simulink library "tqd"  (R2021b)
settings: Solver=VariableStepAuto  StartTime=0.0  StopTime=10.0  RelTol=1e-3
undefined symbols (not defined in the file): ATQD_AfterTqMinGain_X_Deg, ATQD_APSCreepBaseTqD_X_kph, ATQD_APSCreepBaseTqD_Y_Deg, ATQD_APSCreepBaseTqR_X_kph, ATQD_APSCreepBaseTqR_Y_Deg, ATQD_APSCreepIterm_X_kph, ATQD_APSCreepIterm_Y_kph, ATQD_APSCreepPterm_X_kph, ATQD_APSCreepPterm_Y_kph, ATQD_APSDecReq_X_kph, ATQD_APSDecReq_Y_mps2, ATQD_APSDecReqCMD_X_kph, ATQD_APSDecReqTs_X_pct, ATQD_APSDecTimeGain_X_Deg, ATQD_APSDecTimeGain_Y_s, ATQD_APSReqLowSpd_X_Deg, ATQD_AutoHoldReleaseBPS_X_Deg, ATQD_AWDLoadTrqnsGain_X_kg, ATQD_AWDLoadTrqnsGain_Y_pct, ATQD_BOSEnBPSPosn_X_kph, ATQD_BOSMap_X_rpm, ATQD_BOSMap_Y_pct, ATQD_CreepBaseTqD_X_kph, ATQD_CreepBaseTqD_Y_Deg, ATQD_CreepBaseTqR_X_kph, ATQD_CreepBaseTqR_Y_Deg, ATQD_CreepBPSDisPosn_X_Deg, ATQD_CreepBPSDisPosnR_X_Deg, ATQD_CreepBPSEnPosn_X_Deg, ATQD_CreepBPSEnPosnR_X_Deg, ATQD_CreepDeltaTq_X_kph, ATQD_CreepIterm_X_kph, ATQD_CreepIterm_Y_kph, ATQD_CreepItermMaxLimit_X_pct, ATQD_CreepPreloadTime_X_kph, ATQD_CreepPreloadTq_X_kph, ATQD_CreepPreloadTq_Y_s, ATQD_CreepProtTq_X_Deg, ATQD_CreepPterm_X_kph, ATQD_CreepPterm_Y_kph, ATQD_CreepRrTqSpRat_X_rpm, ATQD_CreepRrTqSpRat_Y_Nm, ATQD_CreepTargetSpdD_X_pct, ATQD_CreepTargetSpdR_X_pct, ATQD_ECOTqMapD_X_rpm, ATQD_ECOTqMapD_Y_pct, ATQD_EMTqMapD_X_rpm, ATQD_EMTqMapD_Y_pct, ATQD_EOPDTqMapDCon_X_rpm, ATQD_EOPDTqMapDCon_Y_Deg, ATQD_EscapeModePedTq_X_pct, ATQD_EscapeModePedTq_Y_rpm, ATQD_EscapeModePedTqFr_X_pct, ATQD_EscapeModePedTqFr_Y_rpm, ATQD_EstInitVehWeight_X_c, ATQD_FAfterTqCMDGain_X_rpm, ATQD_FAfterTqCMDGain_Y_pct, ATQD_FrLossMAPLowV_X_rpm, ATQD_FrLossMAPLowV_Y_Nm, ATQD_FrMotActReduce_X_rpm ... (+772)
libraries: simulink x211, hcu_lib x179, tqr x3
(part 9 of 28)

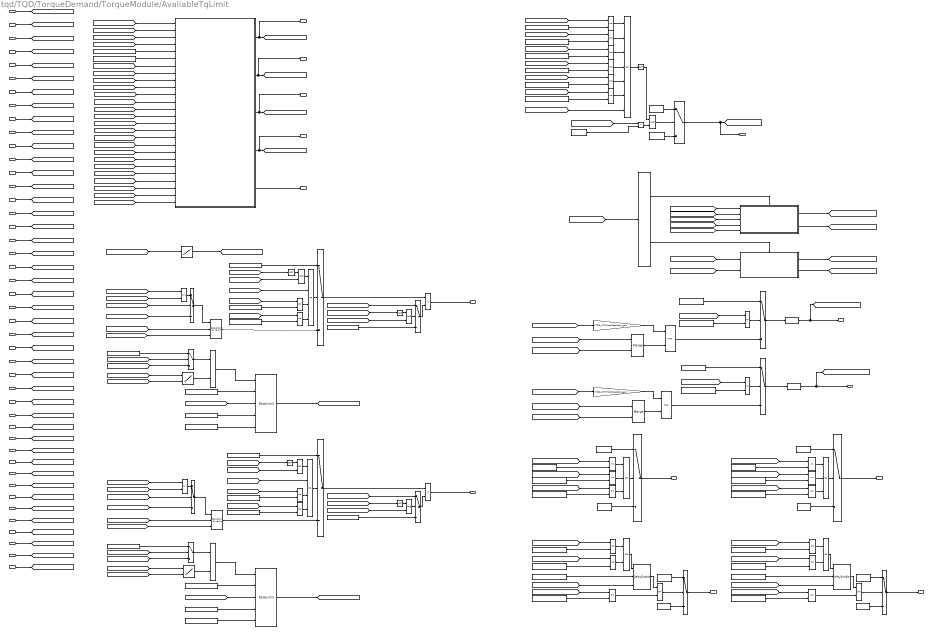
== system tqd/TQD/TorqueDemand/TorqueModule/AvaliableTqLimit ==
  note: Avaiable Torque for B-type Regen
  note: Available Torque Calculation
  note: A-regen activation judgment
  VTQD_FrShaftSpd_rpm : Inport
  VTQD_RrShaftSpd_rpm : Inport  Port=2
  VINP_HVBPwrAvailDchrg_kw : Inport  Port=3
  VINP_HVBPwrAvailChrg_kw : Inport  Port=4
  VTQD_CoordWhlTqDemFr_Nm : Inport  Port=5
  VTQD_CoordWhlTqDemRr_Nm : Inport  Port=6
  VTQD_FrEDUSpRat_rat : Inport  Port=7
  VTQD_RrEDUSpRat_rat : Inport  Port=8
  VTQD_TqSourceFr_enum : Inport  Port=9
  VTQD_TqSourceRr_enum : Inport  Port=10
  VTQD_DriverWhlTqDemFr_Nm : Inport  Port=11
  VTQD_DriverWhlTqDemRr_Nm : Inport  Port=12
  VINP_FrRegenAvailTq_Nm : Inport  Port=13
  VINP_RrRegenAvailTq_Nm : Inport  Port=14
  VTQD_DriverWhlTqDem_Nm : Inport  Port=15
  VINP_FrMotorAvailTq_Nm : Inport  Port=16
  VINP_RrMotorAvailTq_Nm : Inport  Port=17
  VTQD_CreepEnable_flg : Inport  Port=18
  VVMC_ADASActive_flg : Inport  Port=19
  VTQD_DriveProtRemove_flg : Inport  Port=20
  VINP_FrPTCSActive_flg : Inport  Port=21
  VINP_RrPTCSActive_flg : Inport  Port=22
  VINP_FrntAxlTrqReqDrv_Nm : Inport  Port=23
  VINP_RearAxlTrqReqDrv_Nm : Inport  Port=24
  VTQD_VehActSpd_kph : Inport  Port=25
  VTQD_PreLoadPreEn_flg : Inport  Port=26
  VVMC_CAASActive_flg : Inport  Port=27
  VTQD_GearActualPosn_enum : Inport  Port=28
  VTQD_FrontSlideRate_pct : Inport  Port=29
  VTQD_RearSlideRate_pct : Inport  Port=30
  VINP_IVISnowModeCmd_flg : Inport  Port=31
  VTQD_IVIRockModeEn_flg : Inport  Port=32
  task_time_s : Inport  Port=33
  VINP_HVBattSOC_pct : Inport  Port=34
  VPMM_DrivetrainSelect_enum : Inport  Port=35
  VINP_VehicleType_enum : Inport  Port=36
  VVMC_EstSlope_Deg : Inport  Port=37
  VINP_FrMCUDCBusVolt_V : Inport  Port=38
  VINP_RrMCUDCBusVolt_V : Inport  Port=39
  VINP_FrMCUTemp_C : Inport  Port=40
  VINP_FrTMTemp_C : Inport  Port=41
  VINP_RrMCUTemp_C : Inport  Port=42
  VINP_RrTMTemp_C : Inport  Port=43
  VTQD_ActAPSPosn_pct : Inport  Port=44
  AND{,1..3} (4 alike) : Logic  AllPortsSameDT=off  OutDataTypeStr=boolean
  Constant{,4,7,37,44} (5 alike) : Constant  Value=FALSE
  Constant1 : Constant  Value=ENUM_TQSOURCE_CC
  Constant10 : Constant  Value=ENUM_TQSOURCE_APS
  Constant11 : Constant  Value=ENUM_TQSOURCE_CC
  Constant12 : Constant  Value=ENUM_TQSOURCE_APS
  Constant13 : Constant  Value=ENUM_TQSOURCE_ADAS
  Constant{14,16..17,19..20,33,48} (7 alike) : Constant  Value=ZERO_FLOAT
  Constant15 : Constant  Value=KTQD_AvailBrkRgnTqSpd_kph
  Constant18 : Constant  Value=KTQD_AvailBrkRgnTqSpd_kph
  Constant2 : Constant  Value=KTQD_FrBatapCont_factor
  Constant{21,23,35,42} (4 alike) : Constant  Value=ENUM_GEARACTUALPOSN_N
  Constant{22,24,36,43} (4 alike) : Constant  Value=ENUM_GEARACTUALPOSN_P
  Constant{25..27,30,51..52} (6 alike) : Constant  Value=ONE_FLOAT
  Constant28 : Constant  Value=KTQD_FAfterTqCMDGainInc_c
  Constant29 : Constant  Value=KTQD_FAfterTqCMDGainDec_c
  Constant{3,6,8,38,45} (5 alike) : Constant  Value=TRUE
  Constant31 : Constant  Value=KTQD_RAfterTqCMDGainInc_c
  Constant32 : Constant  Value=KTQD_RAfterTqCMDGainDec_c
  Constant34 : Constant  Value=KTQD_AvailBRgnTqVSOC_pct
  Constant39 : Constant  Value=ENUM_DRIVETRAIN_RWD
  Constant40 : Constant  Value=ENUM_DRIVETRAIN_RWD
  Constant41 : Constant  Value=KTQD_BRgnPermDisDelay_s
  Constant46 : Constant  Value=ENUM_DRIVETRAIN_FWD
  Constant47 : Constant  Value=KTQD_BRgnPermDisDelay_s
  Constant49 : Constant  Value=KTQD_AvailBRgnTqVSOC_pct
  Constant5 : Constant  Value=KTQD_RrBatapCont_factor
  Constant50 : Constant  Value=ENUM_DRIVETRAIN_FWD
  Constant9 : Constant  Value=ENUM_TQSOURCE_ADAS
  Data Type Conversion : DataTypeConversion  OutDataTypeStr=single
  Data Type Conversion1 : DataTypeConversion  OutDataTypeStr=single
  DelayEnable : hcu_lib/Basic_Blocks/DelayEnable
  DelayEnable1 : hcu_lib/Basic_Blocks/DelayEnable
  Equal{,1..17} (18 alike) : RelationalOperator  Operator===  OutDataTypeStr=boolean  RndMeth=Simplest
  Gain : Gain  Gain=KTQD_FrTMTotalGearRatio_gain
  Gain1 : Gain  Gain=KTQD_RrTMTotalGearRatio_gain
  If : If  IfExpression=u1 ~= 0
  If Action Subsystem1 : Subsystem  TreatAsAtomicUnit=on
  If Action Subsystem2 : Subsystem  TreatAsAtomicUnit=on
  Logical Operator : Logic  Operator=OR  Inputs=7  AllPortsSameDT=off  OutDataTypeStr=boolean
  Logical Operator1 : Logic  AllPortsSameDT=off  OutDataTypeStr=boolean
  Logical Operator2 : Logic  Operator=NOT  AllPortsSameDT=off  OutDataTypeStr=boolean
  MTQD_AfterTqMinGain_Y_c : Lookup_n-D  NumberOfTableDimensions=1  BreakpointsForDimension1=ATQD_AfterTqMinGain_X_Deg  Table=MTQD_AfterTqMinGain_Y_c  InternalRulePriority=Speed  RndMeth=Simplest  InputSameDT=on
  MTQD_FAfterTqCMDGain_Z_c : Lookup_n-D  BreakpointsForDimension1=ATQD_FAfterTqCMDGain_Y_pct  BreakpointsForDimension2=ATQD_FAfterTqCMDGain_X_rpm  Table=MTQD_FAfterTqCMDGain_Z_c  InternalRulePriority=Speed  RndMeth=Simplest  InputSameDT=on
      settings: InputPortMap=u0,u1
  MTQD_RAfterTqCMDGain_Z_c : Lookup_n-D  BreakpointsForDimension1=ATQD_FAfterTqCMDGain_Y_pct  BreakpointsForDimension2=ATQD_FAfterTqCMDGain_X_rpm  Table=MTQD_RAfterTqCMDGain_Z_c  InternalRulePriority=Speed  RndMeth=Simplest  InputSameDT=on
      settings: InputPortMap=u0,u1
  Max{,1..3} (4 alike) : MinMax  Function=max  Inputs=2
  Merge : Merge
  Merge1 : Merge
  Min : MinMax  Inputs=2
  Min1 : MinMax  Inputs=2
  NOT{,1..3} (4 alike) : Logic  Operator=NOT  AllPortsSameDT=off  OutDataTypeStr=boolean
  OR : Logic  Operator=OR  Inputs=4  AllPortsSameDT=off  OutDataTypeStr=boolean
  OR1 : Logic  Operator=OR  Inputs=4  AllPortsSameDT=off  OutDataTypeStr=boolean
  OR2 : Logic  Operator=OR  Inputs=3  AllPortsSameDT=off  OutDataTypeStr=boolean
  OR{3..6} (4 alike) : Logic  Operator=OR  AllPortsSameDT=off  OutDataTypeStr=boolean
  OR7 : Logic  Operator=OR  Inputs=3  AllPortsSameDT=off  OutDataTypeStr=boolean
  Product : Product
  Product1 : Product
  RateLimit : hcu_lib/Basic_Blocks/RateLimit
  RateLimit1 : hcu_lib/Basic_Blocks/RateLimit
  Relational Operator : RelationalOperator  Operator=<  OutDataTypeStr=boolean  RndMeth=Simplest
  Relational Operator1 : RelationalOperator  Operator=<=  OutDataTypeStr=boolean  RndMeth=Simplest
  Relational Operator2 : RelationalOperator  Operator=<=  OutDataTypeStr=boolean  RndMeth=Simplest
  Relational Operator{3..6} (4 alike) : RelationalOperator  OutDataTypeStr=boolean  RndMeth=Simplest
  Saturation Dynamic : simulink/Discontinuities/Saturation Dynamic  OutMin=[]  OutMax=[]  OutDataTypeStr=Inherit: Same as second input  OutDataType=fixdt(1, 16)  OutScaling=2^-10  DoSatur=off
  Saturation Dynamic1 : simulink/Discontinuities/Saturation Dynamic  OutMin=[]  OutMax=[]  OutDataTypeStr=Inherit: Same as second input  OutDataType=fixdt(1, 16)  OutScaling=2^-10  DoSatur=off
  Switch{,1,5..14} (12 alike) : Switch  Criteria=u2 > Threshold
  Switch2 : Switch  Criteria=u2 ~= 0
  Switch3 : Switch  Criteria=u2 ~= 0
  Switch4 : Switch  Criteria=u2 ~= 0
  TorqueCapacityCalcalation : Subsystem
  VTQD_AfterAvailableTqDemFr_Nm : Outport
  VTQD_AfterAvailableTqDemRr_Nm : Outport  Port=2
  VTQD_FrEDUAvailBrkRgnTq_Nm : Outport  Port=3
  VTQD_RrEDUAvailBrkRgnTq_Nm : Outport  Port=4
  VTQD_FrRgnDecrSta_flg : Outport  Port=5
  VTQD_RrRgnDecrSta_flg : Outport  Port=6
  VTQD_FrRgnPermSta_flg : Outport  Port=7
  VTQD_RrRgnPermSta_flg : Outport  Port=8
  VTQD_ARegenActive_flg : Outport  Port=9
  VTQD_WhlTqCapGenFr_Nm : Outport  Port=10
  VTQD_WhlTqCapGenRr_Nm : Outport  Port=11
  VTQD_WhlTqCapMotFr_Nm : Outport  Port=12
  VTQD_WhlTqCapMotRr_Nm : Outport  Port=13
  VTQD_MotorLossTotal_kw : Outport  Port=14
  wires:
  VINP_FrRegenAvailTq_Nm/1 -> [VINP_FrRegenAvailTq_Nm]
  VINP_RrRegenAvailTq_Nm/1 -> [VINP_RrRegenAvailTq_Nm]
  Merge1/1 -> Max1/2
  [VINP_RrRegenAvailTq_Nm] -> Gain1/1
  Gain1/1 -> Max1/1
  Gain/1 -> Max/1
  Merge/1 -> Max/2
  [VINP_FrRegenAvailTq_Nm] -> Gain/1
  [VTQD_ARegenActive_flg] -> If/1
  Switch1/1 -> VTQD_RrRgnDecrSta_flg/1
  Switch/1 -> VTQD_FrRgnDecrSta_flg/1
  Constant3/1 -> Switch/3
  Constant/1 -> Switch/1
  If/2 -> If Action Subsystem2/Action
  If/1 -> If Action Subsystem1/Action
  Data Type Conversion1/1 -> VTQD_RrEDUAvailBrkRgnTq_Nm/1, [VTQD_RrEDUAvailBrkRgnTq_Nm]  "VTQD_RrEDUAvailBrkRgnTq_Nm"
  Data Type Conversion/1 -> VTQD_FrEDUAvailBrkRgnTq_Nm/1, [VTQD_FrEDUAvailBrkRgnTq_Nm]  "VTQD_FrEDUAvailBrkRgnTq_Nm"
  TorqueCapacityCalcalation/4(VTQD_WhlTqCapGenRr_Nm) -> VTQD_WhlTqCapGenRr_Nm/1, [VTQD_WhlTqCapGenRr_Nm]
  TorqueCapacityCalcalation/2(VTQD_WhlTqCapMotRr_Nm) -> VTQD_WhlTqCapMotRr_Nm/1, [VTQD_WhlTqCapMotRr_Nm]
  VTQD_RrShaftSpd_rpm/1 -> [VTQD_RrShaftSpd_rpm]
  [VTQD_RrEDUSpRat_rat] -> TorqueCapacityCalcalation/8(VTQD_RrEDUSpRat_rat)
  [VTQD_FrEDUSpRat_rat] -> TorqueCapacityCalcalation/7(VTQD_FrEDUSpRat_cmd)
  Constant5/1 -> TorqueCapacityCalcalation/6(KTQD_RrBatapCont_factor)
  [VTQD_RrShaftSpd_rpm] -> TorqueCapacityCalcalation/2(VTQD_RrShaftSpd_rpm)
  Constant2/1 -> TorqueCapacityCalcalation/5(KTQD_FrBatapCont_factor)
  [VINP_HVBPwrAvailChrg_kw] -> TorqueCapacityCalcalation/4(VINP_HVBPwrAvailChrg_kw)
  [VINP_HVBPwrAvailDchrg_kw] -> TorqueCapacityCalcalation/3(VINP_HVBPwrAvailDchrg_kw)
  [VTQD_FrShaftSpd_rpm] -> TorqueCapacityCalcalation/1(VTQD_FrShaftSpd_rpm)
  TorqueCapacityCalcalation/3(VTQD_WhlTqCapGenFr_Nm) -> VTQD_WhlTqCapGenFr_Nm/1, [VTQD_WhlTqCapGenFr_Nm]
  If Action Subsystem2/2(VTQD_AvailTqNoARgnRr_Nm) -> [VTQD_AvailTqNoARgnRr_Nm]
  If Action Subsystem2/1(VTQD_AvailTqNoARgnFr_Nm) -> [VTQD_AvailTqNoARgnFr_Nm]
  [VTQD_WhlTqCapGenRr_Nm] -> If Action Subsystem2/2(VTQD_WhlTqCapGenR_Nm)
  [VTQD_WhlTqCapGenFr_Nm] -> If Action Subsystem2/1(VTQD_WhlTqCapGenF_Nm)
  [VTQD_WhlTqCapGenRr_Nm] -> If Action Subsystem1/2(VTQD_WhlTqCapGenR_Nm)
  [VTQD_WhlTqCapGenFr_Nm] -> If Action Subsystem1/1(VTQD_WhlTqCapGenF_Nm)
  [VTQD_DriverWhlTqDemRr_Nm] -> If Action Subsystem1/4(VTQD_DriverWhlTqDemRr_Nm)
  [VTQD_DriverWhlTqDemFr_Nm] -> If Action Subsystem1/3(VTQD_DriverWhlTqDemFr_Nm)
  VTQD_DriverWhlTqDemRr_Nm/1 -> [VTQD_DriverWhlTqDemRr_Nm]
  VTQD_DriverWhlTqDemFr_Nm/1 -> [VTQD_DriverWhlTqDemFr_Nm]
  VTQD_TqSourceFr_enum/1 -> [VTQD_TqSourceFr_enum]
  VTQD_RrEDUSpRat_rat/1 -> [VTQD_RrEDUSpRat_rat]
  VTQD_FrEDUSpRat_rat/1 -> [VTQD_FrEDUSpRat_rat]
  VTQD_CoordWhlTqDemRr_Nm/1 -> [VTQD_CoordWhlTqDemRr_Nm]
  VTQD_CoordWhlTqDemFr_Nm/1 -> [VTQD_CoordWhlTqDemFr_Nm]
  VINP_HVBPwrAvailDchrg_kw/1 -> [VINP_HVBPwrAvailDchrg_kw]
  VTQD_FrShaftSpd_rpm/1 -> [VTQD_FrShaftSpd_rpm]
  VINP_HVBPwrAvailChrg_kw/1 -> [VINP_HVBPwrAvailChrg_kw]
  VTQD_TqSourceRr_enum/1 -> [VTQD_TqSourceRr_enum]
  Switch2/1 -> [VTQD_ARegenActive_flg], VTQD_ARegenActive_flg/1  "VTQD_ARegenActive_flg"
  VTQD_DriverWhlTqDem_Nm/1 -> [VTQD_DriverWhlTqDem_Nm]
  VINP_RrMotorAvailTq_Nm/1 -> [VINP_RrMotorAvailTq_Nm]
  VINP_FrMotorAvailTq_Nm/1 -> [VINP_FrMotorAvailTq_Nm]
  [VINP_FrMotorAvailTq_Nm] -> TorqueCapacityCalcalation/9(VINP_FrMotorAvailTq_Nm)
  [VINP_RrMotorAvailTq_Nm] -> TorqueCapacityCalcalation/10(VINP_RrMotorAvailTq_Nm)
  VTQD_CreepEnable_flg/1 -> [VTQD_CreepEnable_flg]
  [VTQD_TqSourceFr_enum] -> Equal/1
  Constant1/1 -> Equal/2
  Constant9/1 -> Equal1/2
  [VTQD_TqSourceFr_enum] -> Equal1/1
  [VTQD_TqSourceFr_enum] -> Equal2/1
  Constant10/1 -> Equal2/2
  Constant12/1 -> Equal5/2
  [VTQD_TqSourceRr_enum] -> Equal5/1
  [VTQD_TqSourceRr_enum] -> Equal4/1
  Constant13/1 -> Equal4/2
  Constant11/1 -> Equal3/2
  [VTQD_TqSourceRr_enum] -> Equal3/1
  Equal5/1 -> Logical Operator/6
  Equal4/1 -> Logical Operator/5
  Equal3/1 -> Logical Operator/4
  Equal2/1 -> Logical Operator/3
  Equal1/1 -> Logical Operator/2
  Equal/1 -> Logical Operator/1
  [VTQD_CreepEnable_flg] -> Logical Operator/7
  Logical Operator/1 -> Logical Operator2/1
  Logical Operator1/1 -> Switch2/2
  [VTQD_DriverWhlTqDem_Nm] -> Relational Operator/1
  Relational Operator/1 -> Logical Operator1/2
  Constant14/1 -> Relational Operator/2
  Constant7/1 -> Switch2/3
  Constant8/1 -> Switch2/1
  Logical Operator2/1 -> Logical Operator1/1
  Constant17/1 -> Switch3/1
  Relational Operator1/1 -> Switch3/2
  Constant15/1 -> Relational Operator1/2
  Max/1 -> Switch3/3
  Switch3/1 -> Data Type Conversion/1
  Constant20/1 -> Switch4/1
  Max1/1 -> Switch4/3
  Relational Operator2/1 -> Switch4/2
  Constant18/1 -> Relational Operator2/2
  Switch4/1 -> Data Type Conversion1/1
  VVMC_ADASActive_flg/1 -> [VVMC_ADASActive_flg]
  [VVMC_ADASActive_flg] -> If Action Subsystem1/5(VVMC_ADASActive_flg)
  [VTQD_AvailTqNoARgnRr_Nm] -> Merge1/2
  [VTQD_AvailTqWithARgnRr_Nm] -> Merge1/1
  [VTQD_AvailTqNoARgnFr_Nm] -> Merge/2
  [VTQD_AvailTqWithARgnFr_Nm] -> Merge/1
  Constant16/1 -> Switch5/1
  Saturation Dynamic/1 -> Switch5/3
  Constant19/1 -> Switch6/1
  Saturation Dynamic1/1 -> Switch6/3
  VTQD_DriveProtRemove_flg/1 -> [VTQD_DriveProtRemove_flg]
  [VTQD_CoordWhlTqDemFr_Nm] -> Saturation Dynamic/2
  Switch7/1 -> Saturation Dynamic/1  "VTQD_FrAvailableTqUpLimt_Nm"
  [VTQD_WhlTqCapMotFr_Nm] -> Switch7/3
  [VINP_FrPTCSActive_flg] -> Switch7/2
  VINP_RearAxlTrqReqDrv_Nm/1 -> [VINP_RearAxlTrqReqDrv_Nm]
  VINP_FrntAxlTrqReqDrv_Nm/1 -> [VINP_FrntAxlTrqReqDrv_Nm]
  VINP_RrPTCSActive_flg/1 -> [VINP_RrPTCSActive_flg]
  VINP_FrPTCSActive_flg/1 -> [VINP_FrPTCSActive_flg]
  [VINP_RrPTCSActive_flg] -> Switch8/2
  [VTQD_WhlTqCapMotRr_Nm] -> Switch8/3
  Switch8/1 -> Saturation Dynamic1/1  "VTQD_RrAvailableTqUpLimt_Nm"
  [VTQD_CoordWhlTqDemRr_Nm] -> Saturation Dynamic1/2
  [VTQD_WhlTqCapMotFr_Nm] -> Min/2
  Min/1 -> Switch7/1
  [VINP_FrntAxlTrqReqDrv_Nm] -> Min/1
  [VTQD_WhlTqCapMotRr_Nm] -> Min1/2
  Min1/1 -> Switch8/1
  [VINP_RearAxlTrqReqDrv_Nm] -> Min1/1
  VTQD_VehActSpd_kph/1 -> [VTQD_VehActSpd_kph]
  [VTQD_VehActSpd_kph] -> Relational Operator1/1
  [VTQD_VehActSpd_kph] -> Relational Operator2/1
  [VTQD_WhlTqCapGenFr_Nm] -> Saturation Dynamic/3
  [VTQD_WhlTqCapGenRr_Nm] -> Saturation Dynamic1/3
  VVMC_CAASActive_flg/1 -> [VVMC_CAASActive_flg]
  VTQD_PreLoadPreEn_flg/1 -> [VTQD_PreLoadPreEn_flg]
  OR/1 -> Switch5/2
  AND/1 -> OR/1
  [VTQD_DriveProtRemove_flg] -> OR/2
  NOT/1 -> AND/1
  [VTQD_PreLoadPreEn_flg] -> NOT/1
  [VVMC_CAASActive_flg] -> AND/2
  NOT1/1 -> AND1/1
  AND1/1 -> OR1/1
  [VVMC_CAASActive_flg] -> AND1/2
  [VTQD_PreLoadPreEn_flg] -> NOT1/1
  [VTQD_DriveProtRemove_flg] -> OR1/2
  If Action Subsystem1/1(VTQD_AvailTqWithARgnFr_Nm) -> [VTQD_AvailTqWithARgnFr_Nm]
  If Action Subsystem1/2(VTQD_AvailTqWithARgnRr_Nm) -> [VTQD_AvailTqWithARgnRr_Nm]
  [VINP_RrRegenAvailTq_Nm] -> TorqueCapacityCalcalation/12(VINP_RrRegenAvailTq_Nm)
  [VINP_FrRegenAvailTq_Nm] -> TorqueCapacityCalcalation/11(VINP_FrRegenAvailTq_Nm)
  [VTQD_GearActualPosn_enum] -> TorqueCapacityCalcalation/13(VTQD_GearActualPosn_enum)
  VTQD_GearActualPosn_enum/1 -> [VTQD_GearActualPosn_enum]
  TorqueCapacityCalcalation/1(VTQD_WhlTqCapMotFr_Nm) -> VTQD_WhlTqCapMotFr_Nm/1, [VTQD_WhlTqCapMotFr_Nm]
  Equal6/1 -> OR/3
  Equal7/1 -> OR/4
  [VTQD_GearActualPosn_enum] -> Equal6/1
  Constant21/1 -> Equal6/2
  [VTQD_GearActualPosn_enum] -> Equal7/1
  Constant22/1 -> Equal7/2
  Constant23/1 -> Equal8/2
  Constant24/1 -> Equal9/2
  [VTQD_GearActualPosn_enum] -> Equal8/1
  Equal9/1 -> OR1/4
  [VTQD_GearActualPosn_enum] -> Equal9/1
  Equal8/1 -> OR1/3
  OR1/1 -> Switch6/2
  VTQD_RearSlideRate_pct/1 -> [VTQD_RearSlideRate_pct]
  VTQD_FrontSlideRate_pct/1 -> [VTQD_FrontSlideRate_pct]
  [VTQD_FrontSlideRate_pct] -> MTQD_FAfterTqCMDGain_Z_c/1
  [VTQD_FrShaftSpd_rpm] -> MTQD_FAfterTqCMDGain_Z_c/2
  VINP_IVISnowModeCmd_flg/1 -> [VINP_IVISnowModeCmd_flg]
  VTQD_IVIRockModeEn_flg/1 -> [VTQD_IVIRockModeEn_flg]
  [VTQD_RrShaftSpd_rpm] -> MTQD_RAfterTqCMDGain_Z_c/2
  [VTQD_RearSlideRate_pct] -> MTQD_RAfterTqCMDGain_Z_c/1
  AND2/1 -> Switch9/2
  [VTQD_FAfterTqCMDGain_c] -> Switch9/1
  Switch5/1 -> Product/1
  Switch9/1 -> Product/2
  Product/1 -> VTQD_AfterAvailableTqDemFr_Nm/1  "VTQD_AfterAvailableTqDemFr_Nm"
  NOT2/1 -> AND2/1
  [VINP_IVISnowModeCmd_flg] -> AND2/2
  [VTQD_IVIRockModeEn_flg] -> NOT2/1
  Constant25/1 -> Switch9/3
  [VTQD_RAfterTqCMDGain_c] -> Switch10/1
  NOT3/1 -> AND3/1
  AND3/1 -> Switch10/2
  Switch10/1 -> Product1/2
  Constant26/1 -> Switch10/3
  [VTQD_IVIRockModeEn_flg] -> NOT3/1
  [VINP_IVISnowModeCmd_flg] -> AND3/2
  Switch6/1 -> Product1/1
  Product1/1 -> VTQD_AfterAvailableTqDemRr_Nm/1  "VTQD_AfterAvailableTqDemRr_Nm"
  RateLimit/1 -> [VTQD_FAfterTqCMDGain_c]  "VTQD_FAfterTqCMDGain_c"
  Constant27/1 -> RateLimit/2
  task_time_s/1 -> [task_time_s]
  [task_time_s] -> RateLimit/3
  Constant28/1 -> RateLimit/4
  Constant29/1 -> RateLimit/5
  Constant31/1 -> RateLimit1/4
  [task_time_s] -> RateLimit1/3
  Constant30/1 -> RateLimit1/2
  Constant32/1 -> RateLimit1/5
  RateLimit1/1 -> [VTQD_RAfterTqCMDGain_c]  "VTQD_RAfterTqCMDGain_c"
  VINP_HVBattSOC_pct/1 -> [VINP_HVBattSOC_pct]
  OR2/1 -> Switch/2
  Relational Operator3/1 -> OR2/1
  [VTQD_FrEDUAvailBrkRgnTq_Nm] -> Relational Operator3/1
  Constant33/1 -> Relational Operator3/2
  Relational Operator4/1 -> OR2/2
  [VINP_HVBattSOC_pct] -> Relational Operator4/1
  Constant34/1 -> Relational Operator4/2
  [VTQD_GearActualPosn_enum] -> Equal10/1
  Constant35/1 -> Equal10/2
  Equal10/1 -> OR3/1
  Constant36/1 -> Equal11/2
  [VTQD_GearActualPosn_enum] -> Equal11/1
  Equal11/1 -> OR3/2
  OR3/1 -> DelayEnable/1
  Constant37/1 -> Switch11/1
  Constant38/1 -> Switch11/3
  Switch11/1 -> VTQD_FrRgnPermSta_flg/1
  VPMM_DrivetrainSelect_enum/1 -> [VPMM_DrivetrainSelect_enum]
  Equal12/1 -> OR2/3
  [VPMM_DrivetrainSelect_enum] -> Equal12/1
  Constant39/1 -> Equal12/2
  DelayEnable/1 -> OR4/1
  Constant40/1 -> Equal13/2
  [VPMM_DrivetrainSelect_enum] -> Equal13/1
  Equal13/1 -> OR4/2
  OR4/1 -> Switch11/2
  [task_time_s] -> DelayEnable/3
  Constant41/1 -> DelayEnable/2
  OR6/1 -> Switch12/2
  Constant45/1 -> Switch12/3
  [VTQD_GearActualPosn_enum] -> Equal15/1
  Constant47/1 -> DelayEnable1/2
  Constant43/1 -> Equal15/2
  Equal14/1 -> OR5/1
  [task_time_s] -> DelayEnable1/3
  DelayEnable1/1 -> OR6/1
  Equal15/1 -> OR5/2
  Equal16/1 -> OR6/2
  OR5/1 -> DelayEnable1/1
  Constant46/1 -> Equal16/2
  Constant42/1 -> Equal14/2
  Constant44/1 -> Switch12/1
  [VPMM_DrivetrainSelect_enum] -> Equal16/1
  [VTQD_GearActualPosn_enum] -> Equal14/1
  Switch12/1 -> VTQD_RrRgnPermSta_flg/1
  [VINP_HVBattSOC_pct] -> Relational Operator6/1
  Relational Operator6/1 -> OR7/2
  Constant49/1 -> Relational Operator6/2
  Constant4/1 -> Switch1/1
  Relational Operator5/1 -> OR7/1
  Constant6/1 -> Switch1/3
  Constant50/1 -> Equal17/2
  Equal17/1 -> OR7/3
  [VPMM_DrivetrainSelect_enum] -> Equal17/1
  Constant48/1 -> Relational Operator5/2
  [VTQD_RrEDUAvailBrkRgnTq_Nm] -> Relational Operator5/1
  OR7/1 -> Switch1/2
  VINP_VehicleType_enum/1 -> [VINP_VehicleType_enum]
  [VINP_VehicleType_enum] -> TorqueCapacityCalcalation/14(VINP_VehicleType_enum)
  VVMC_EstSlope_Deg/1 -> [VVMC_EstSlope_Deg]
  [VVMC_EstSlope_Deg] -> MTQD_AfterTqMinGain_Y_c/1
  MTQD_AfterTqMinGain_Y_c/1 -> [VTQD_AfterTqMinGain_c]  "VTQD_AfterTqMinGain_c"
  MTQD_FAfterTqCMDGain_Z_c/1 -> Max2/2
  Max2/1 -> RateLimit/1
  Switch13/1 -> Max2/1
  [VTQD_AfterTqMinGain_c] -> Switch13/3
  [VINP_FrPTCSActive_flg] -> Switch13/2
  Constant51/1 -> Switch13/1
  Switch14/1 -> Max3/1
  [VTQD_AfterTqMinGain_c] -> Switch14/3
  Constant52/1 -> Switch14/1
  [VINP_RrPTCSActive_flg] -> Switch14/2
  MTQD_RAfterTqCMDGain_Z_c/1 -> Max3/2
  Max3/1 -> RateLimit1/1
  [VTQD_CoordWhlTqDemFr_Nm] -> TorqueCapacityCalcalation/15(VTQD_CoordWhlTqDemFr_Nm)
  [VTQD_CoordWhlTqDemRr_Nm] -> TorqueCapacityCalcalation/16(VTQD_CoordWhlTqDemRr_Nm)
  [VINP_FrMCUDCBusVolt_V] -> TorqueCapacityCalcalation/17(VINP_FrMCUDCBusVolt_V)
  [VPMM_DrivetrainSelect_enum] -> TorqueCapacityCalcalation/19(VPMM_DrivetrainSelect_enum)
  [VINP_RrMCUDCBusVolt_V] -> TorqueCapacityCalcalation/18(VINP_RrMCUDCBusVolt_V)
  VINP_RrMCUDCBusVolt_V/1 -> [VINP_RrMCUDCBusVolt_V]
  VINP_FrMCUDCBusVolt_V/1 -> [VINP_FrMCUDCBusVolt_V]
  VINP_FrMCUTemp_C/1 -> [VINP_FrMCUTemp_C]
  VINP_FrTMTemp_C/1 -> [VINP_FrTMTemp_C]
  VINP_RrMCUTemp_C/1 -> [VINP_RrMCUTemp_C]
  VINP_RrTMTemp_C/1 -> [VINP_RrTMTemp_C]
  [VINP_FrMCUTemp_C] -> TorqueCapacityCalcalation/20(VINP_FrMCUTemp_C)
  [VINP_FrTMTemp_C] -> TorqueCapacityCalcalation/21(VINP_FrTMTemp_C)
  [VINP_RrMCUTemp_C] -> TorqueCapacityCalcalation/22(VINP_RrMCUTemp_C)
  [VINP_RrTMTemp_C] -> TorqueCapacityCalcalation/23(VINP_RrTMTemp_C)
  [VTQD_IVIRockModeEn_flg] -> TorqueCapacityCalcalation/24(VTQD_IVIRockModeEn_flg)
  VTQD_ActAPSPosn_pct/1 -> [VTQD_ActAPSPosn_pct]
  [VTQD_ActAPSPosn_pct] -> TorqueCapacityCalcalation/25(VTQD_ActAPSPosn_pct)
  [task_time_s] -> TorqueCapacityCalcalation/26(task_time_s)
  TorqueCapacityCalcalation/5(VTQD_MotorLossTotal_kw) -> VTQD_MotorLossTotal_kw/1

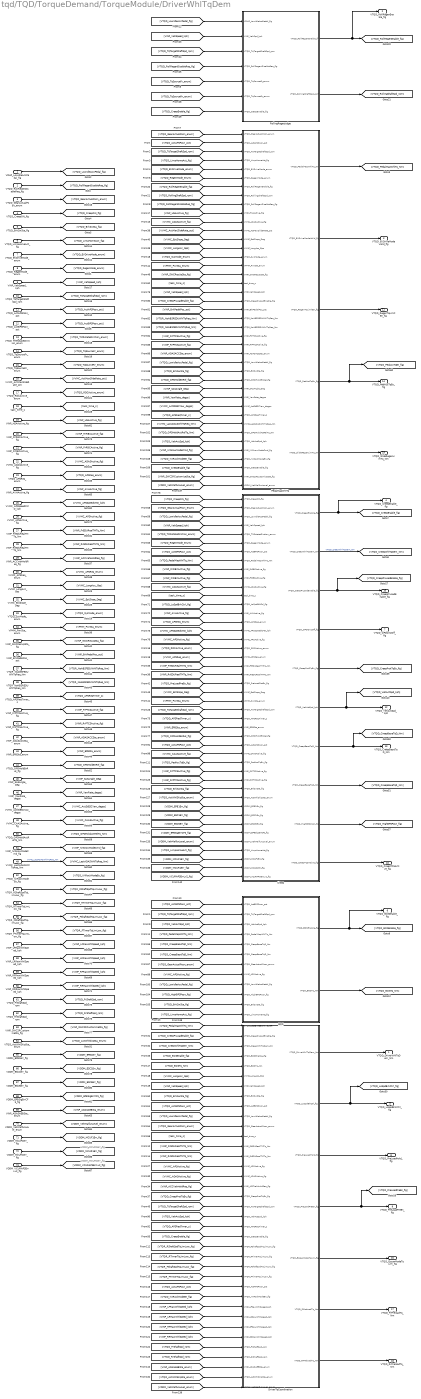
== system tqd/TQD/TorqueDemand/TorqueModule/DriverWhlTqDem ==
  note: VDDM_MCUR1Err_flg
  note: VDDM_MCUR1Err_flg
  VDHP_LowIdleAccPedal_flg : Inport
  VTQD_RollRegenDisableReq_flg : Inport  Port=2
  VTQD_GearActualPosn_enum : Inport  Port=3
  "VTQD_CreepON_flg " : Inport  Port=4
  VTQD_BrkSwSta_flg : Inport  Port=5
  VTQD_LimpHomeAct_flg : Inport  Port=6
  VTQD_EVDriveMode_enum : Inport  Port=7
  VTQD_RegenMode_enum : Inport  Port=8
  VINP_VehSpeed_kph : Inport  Port=9
  VTQD_TqTargetShaftSpd_rpm : Inport  Port=10
  VTQD_ActAPSPosn_pct : Inport  Port=11
  VTQD_ActBPSPosn_pct : Inport  Port=12
  VTQD_TMRotateDirction_enum : Inport  Port=13
  VTQD_TqSourceFr_enum : Inport  Port=14
  VTQD_TqSourceRr_enum : Inport  Port=15
  VVMC_ActMaxSlideRate_pct : Inport  Port=16
  VTQD_RDCActive_enum : Inport  Port=17
  task_time_s : Inport  Port=18
  VINP_HSAActive_flg : Inport  Port=19
  VINP_RrRBCActive_flg : Inport  Port=20
  VINP_FrRBCActive_flg : Inport  Port=21
  VVMC_ADASActive_flg : Inport  Port=22
  VTQD_APSReq_enum : Inport  Port=23
  VINP_AVHActive_flg : Inport  Port=24
  VVMC_APSSpeedCMD_kph : Inport  Port=25
  VVMC_APSActive_flg : Inport  Port=26
  VINP_FrEDURealTMTq_Nm : Inport  Port=27
  VINP_RrEDURealTMTq_Nm : Inport  Port=28
  VINP_ACCVehHoldReq_flg : Inport  Port=29
  VVMC_APSReq_enum : Inport  Port=30
  VVMC_LongAcc_Gps : Inport  Port=31
  VVMC_EstSlope_Deg : Inport  Port=32
  VTQD_SysMode_enum : Inport  Port=33
  VPMM_PwrSta_enum : Inport  Port=34
  VINP_SWCResUpSta_flg : Inport  Port=35
  VINP_BrkPedalPos_pct : Inport  Port=36
  VTQR_NoABSFEDUWhlTqReq_Nm : Inport  Port=37
  VTQR_NoABSREDUWhlTqReq_Nm : Inport  Port=38
  VTQD_APSReqTimer_s : Inport  Port=39
  VINP_FrPTCSActive_flg : Inport  Port=40
  VINP_RrPTCSActive_flg : Inport  Port=41
  VINP_ADASACCSta_enum : Inport  Port=42
  VINP_EPBSta_enum : Inport  Port=43
  VTQD_OPDHoldEnRel_flg : Inport  Port=44
  VINP_SASAngle_Deg : Inport  Port=45
  VINP_YawRate_degps : Inport  Port=46
  VVMC_ActStESCYaw_degps : Inport  Port=47
  VVMC_CAASActive_flg : Inport  Port=48
  VVMC_LastADASWhlTqReq_Nm : Inport  Port=49
  VTQD_OPDHoldActRelTq_Nm : Inport  Port=50
  VINP_IVISnowModeCmd_flg : Inport  Port=51
  VTQD_IVIRockModeEn_flg : Inport  Port=52
  VTQR_RShaftSpdTqLimLow_flg : Inport  Port=53
  VTQR_RTimerTqLimLow_flg : Inport  Port=54
  VTQR_FShaftSpdTqLimLow_flg : Inport  Port=55
  VTQR_FTimerTqLimLow_flg : Inport  Port=56
  VINP_LFRawWhlSpeed_kph : Inport  Port=57
  VINP_LRRawWhlSpeed_kph : Inport  Port=58
  VINP_RFRawWhlSpeed_kph : Inport  Port=59
  VINP_RRRawWhlSpeed_kph : Inport  Port=60
  VTQD_FrShaftSpd_rpm : Inport  Port=61
  VTQD_RrShaftSpd_rpm : Inport  Port=62
  VINP_SWC2RCustomizeSta_flg : Inport  Port=63
  VTQD_ActWhlSkipSta_enum : Inport  Port=64
  VDDM_EPB1Err_flg : Inport  Port=65
  VDDM_ESC1Err_flg : Inport  Port=66
  VDDM_ESC5Err_flg : Inport  Port=67
  VDDM_EPBSigErrCFS_flg : Inport  Port=68
  VINP_ADASAEBSta_enum : Inport  Port=69
  VDDM_VehMalfunLevel_enum : Inport  Port=70
  VDDM_MCUF1Err_flg : Inport  Port=71
  VDDM_MCUR1Err_flg : Inport  Port=72
  VDDM_VCURAPSErrLv2_flg : Inport  Port=73
  BOS : Subsystem
  Creep : Subsystem
  DriverTqCoordination : Subsystem  AncestorBlock=tqd0/TQD/TorqueDemand/TorqueModule/DriverWhlTqDem/DriverTqCoordination
  PedalMapWhlTq : Subsystem
  RollingRegenJudge : Subsystem
  VTQD_DriverWhlTqDem_Nm : Outport
  VTQD_RollRegenEnable_flg : Outport  Port=2
  VTQD_EVDriveModeValid_flg : Outport  Port=3
  VTQD_CreepEnable_flg : Outport  Port=4
  VTQD_LoSpdBrkCtrl_flg : Outport  Port=5
  VTQD_BOSEnable_flg : Outport  Port=6
  VTQD_OPDOn2Off_flg : Outport  Port=7
  VTQD_PreLoadHold_flg : Outport  Port=8
  VTQD_PreLoadPreEn_flg : Outport  Port=9
  VTQD_CreepPrLoadEnable_flg : Outport  Port=10
  VTQD_RegenTqLimitEn_flg : Outport  Port=11
  VTQD_VehActSpd_kph : Outport  Port=12
  VTQD_CreepBaseTqD_Nm : Outport  Port=13
  VTQD_PedAccTqEn_flg : Outport  Port=14
  VTQD_EscapModeTqLim_flg : Outport  Port=15
  VTQD_CreepTCSActive_flg : Outport  Port=16
  VTQD_FrPreloadTq_Nm : Outport  Port=17
  VTQD_RrPreloadTq_Nm : Outport  Port=18
  VTQD_SlideRegenLimTq_Nm : Outport  Port=19
  wires:
  VTQD_BrkSwSta_flg/1 -> [VTQD_BrkSwSta_flg]
  VTQD_ActBPSPosn_pct/1 -> [VTQD_ActBPSPosn_pct]
  VTQD_RegenMode_enum/1 -> [VTQD_RegenMode_enum]
  VINP_VehSpeed_kph/1 -> [VINP_VehSpeed_kph]
  "VTQD_CreepON_flg "/1 -> [VTQD_CreepON_flg]
  PedalMapWhlTq/1(VTQD_PedalMapWhlTq_Nm) -> [VTQD_PedalMapWhlTq_Nm]
  VTQD_LimpHomeAct_flg/1 -> [VTQD_LimpHomeAct_flg]
  VTQD_TqTargetShaftSpd_rpm/1 -> [VTQD_TqTargetShaftSpd_rpm]
  VTQD_EVDriveMode_enum/1 -> [VTQD_EVDriveMode_enum]
  VTQD_ActAPSPosn_pct/1 -> [VTQD_ActAPSPosn_pct]
  VTQD_GearActualPosn_enum/1 -> [VTQD_GearActualPosn_enum]
  VDHP_LowIdleAccPedal_flg/1 -> [VTQD_LowIdleAccPedal_flg]
  BOS/2(VTQD_BOSTq_Nm) -> [VTQD_BOSTq_Nm]
  BOS/1(VTQD_BOSEnable_flg) -> [VTQD_BOSEnable_flg], VTQD_BOSEnable_flg/1
  [VTQD_ActBPSPosn_pct] -> BOS/1(VTQD_ActBPSPosn_pct)
  [VTQD_TqTargetShaftSpd_rpm] -> BOS/2(VTQD_TqTargetShaftSpd_rpm)
  RollingRegenJudge/1(VTQD_RollRegenEnable_flg) -> VTQD_RollRegenEnable_flg/1, [VTQD_RollRegenEnable_flg]
  RollingRegenJudge/2(VTQD_RollingShaftSpd_rpm) -> [VTQD_RollingShaftSpd_rpm]
  VTQD_RollRegenDisableReq_flg/1 -> [VTQD_RollRegenDisableReq_flg]
  PedalMapWhlTq/2(VTQD_EVDriveModeValid_flg) -> VTQD_EVDriveModeValid_flg/1
  VTQD_TMRotateDirction_enum/1 -> [VTQD_TMRotateDirction_enum]
  [VTQD_GearActualPosn_enum] -> PedalMapWhlTq/1(VTQD_GearActualPosn_enum)
  [VTQD_LimpHomeAct_flg] -> PedalMapWhlTq/4(VTQD_LimpHomeAct_flg)
  [VTQD_ActAPSPosn_pct] -> PedalMapWhlTq/2(VTQD_ActAPSPosn_pct)
  [VTQD_TqTargetShaftSpd_rpm] -> PedalMapWhlTq/3(VTQD_TqTargetShaftSpd_rpm)
  [VTQD_RollRegenEnable_flg] -> PedalMapWhlTq/7(VTQD_RollRegenEnable_flg)
  [VTQD_RollingShaftSpd_rpm] -> PedalMapWhlTq/8(VTQD_RollingShaftSpd_rpm)
  [VTQD_RegenMode_enum] -> PedalMapWhlTq/6(VTQD_RegenMode_enum)
  [VTQD_EVDriveMode_enum] -> PedalMapWhlTq/5(VTQD_EVDriveMode_enum)
  [VTQD_TqSourceRr_enum] -> RollingRegenJudge/6(VTQD_TqSourceRr_enum)
  [VINP_VehSpeed_kph] -> RollingRegenJudge/2(VINP_VehSpd_kph)
  [VTQD_TqTargetShaftSpd_rpm] -> RollingRegenJudge/3(VTQD_TqTargetShaftSpd_rpm)
  [VTQD_TqSourceFr_enum] -> RollingRegenJudge/5(VTQD_TqSourceFr_enum)
  [VTQD_CreepEnable_flg] -> RollingRegenJudge/7(VTQD_CreepEnable_flg)
  [VTQD_LowIdleAccPedal_flg] -> RollingRegenJudge/1(VDHP_LowIdleAccPedal_flg)
  VTQD_TqSourceFr_enum/1 -> [VTQD_TqSourceFr_enum]
  VTQD_TqSourceRr_enum/1 -> [VTQD_TqSourceRr_enum]
  VVMC_ActMaxSlideRate_pct/1 -> [VVMC_ActMaxSlideRate_pct]
  VTQD_RDCActive_enum/1 -> [VTQD_RDCActive_enum]
  task_time_s/1 -> [task_time_s]
  [VTQD_RollRegenDisableReq_flg] -> RollingRegenJudge/4(VTQD_RollRegenDisableReq_flg)
  [VINP_VehSpeed_kph] -> DriverTqCoordination/7(VINP_VehSpeed_kph)
  [task_time_s] -> DriverTqCoordination/12(task_time_s)
  [VTQD_LowIdleAccPedal_flg] -> DriverTqCoordination/10(VTQD_LowIdleAccPedal_flg)
  [VTQD_GearActualPosn_enum] -> DriverTqCoordination/11(VTQD_GearActualPosn_enum)
  [VTQD_CreepPrLoadEnable_flg] -> DriverTqCoordination/2(VTQD_CreepPrLoadEnable_flg)
  [VTQD_PedalMapWhlTq_Nm] -> DriverTqCoordination/1(VTQD_PedalMapWhlTq_Nm)
  [VTQD_ActBPSPosn_pct] -> DriverTqCoordination/9(VTQD_ActBPSPosn_pct)
  [VTQD_BOSEnable_flg] -> DriverTqCoordination/4(VTQD_BOSEnable_flg)
  [VTQD_CreepWhlTqDem_Nm] -> DriverTqCoordination/3(VTQD_CreepWhlTqDem_Nm)
  [VTQD_BrkSwSta_flg] -> DriverTqCoordination/8(VTQD_BrkSwSta_flg)
  DriverTqCoordination/2(VTQD_LoSpdBrkCtrl_flg) -> [VTQD_LoSpdBrkCtrl_flg], VTQD_LoSpdBrkCtrl_flg/1
  DriverTqCoordination/1(VTQD_DriverWhlTqDem_Nm) -> VTQD_DriverWhlTqDem_Nm/1
  [VINP_RrRBCActive_flg] -> Creep/9(VINP_RrRBCActive_flg)
  [VINP_FrRBCActive_flg] -> Creep/10(VINP_FrRBCActive_flg)
  [VINP_VehSpeed_kph] -> Creep/4(VINP_VehSpeed_kph)
  [VTQD_ActBPSPosn_pct] -> Creep/7(VTQD_ActBPSPosn_pct)
  [VTQD_TMRotateDirction_enum] -> Creep/5(VTQD_TMRotateDirction_enum)
  [VTQD_CreepON_flg] -> Creep/1(VTQD_CreepON_flg)
  [VTQD_LowIdleAccPedal_flg] -> Creep/3(VTQD_LowIdleAccPedal_flg)
  [VTQD_APSReq_enum] -> Creep/15(VTQD_APSReq_enum)
  [VVMC_APSActive_flg] -> Creep/17(VVMC_APSActive_flg)
  [VTQD_RegenMode_enum] -> Creep/6(VTQD_RegenMode_enum)
  [VINP_AVHActive_flg] -> Creep/14(VINP_AVHActive_flg)
  [VVMC_APSSpeedCMD_kph] -> Creep/16(VVMC_APSSpeedCMD_kph)
  [VTQD_PedalMapWhlTq_Nm] -> Creep/8(VTQD_PedalMapWhlTq_Nm)
  [VTQD_GearActualPosn_enum] -> Creep/2(VTQD_GearActualPosn_enum)
  [VVMC_ADASActive_flg] -> Creep/11(VVMC_ADASActive_flg)
  [task_time_s] -> Creep/12(task_time_s)
  [VTQD_LoSpdBrkCtrl_flg] -> Creep/13(VTQD_LoSpdBrkCtrl_flg)
  Creep/1(VTQD_CreepEnable_flg) -> VTQD_CreepEnable_flg/1, [VTQD_CreepEnable_flg]
  Creep/2(VTQD_CreepWhlTqDem_Nm) -> [VTQD_CreepWhlTqDem_Nm]  "VTQD_CreepWhlTqDem_Nm"
  Creep/3(VTQD_CreepPrLoadEnable_flg) -> [VTQD_CreepPrLoadEnable_flg], VTQD_CreepPrLoadEnable_flg/1
  VVMC_APSActive_flg/1 -> [VVMC_APSActive_flg]
  VTQD_APSReq_enum/1 -> [VTQD_APSReq_enum]
  VVMC_ADASActive_flg/1 -> [VVMC_ADASActive_flg]
  VINP_AVHActive_flg/1 -> [VINP_AVHActive_flg]
  VVMC_APSSpeedCMD_kph/1 -> [VVMC_APSSpeedCMD_kph]
  VINP_FrRBCActive_flg/1 -> [VINP_FrRBCActive_flg]
  VINP_RrRBCActive_flg/1 -> [VINP_RrRBCActive_flg]
  VINP_HSAActive_flg/1 -> [VINP_HSAActive_flg]
  [VTQD_RollRegenDisableReq_flg] -> PedalMapWhlTq/9(VTQD_RollRegenDisableReq_flg)
  [VINP_HSAActive_flg] -> PedalMapWhlTq/10(VINP_HSAActive_flg)
  Creep/4(VTQD_OPDOn2Off_flg) -> VTQD_OPDOn2Off_flg/1
  VINP_RrEDURealTMTq_Nm/1 -> [VINP_RrEDURealTMTq_Nm]
  VINP_FrEDURealTMTq_Nm/1 -> [VINP_FrEDURealTMTq_Nm]
  [VINP_FrEDURealTMTq_Nm] -> DriverTqCoordination/13(VINP_FrEDURealTMTq_Nm)
  [VINP_RrEDURealTMTq_Nm] -> DriverTqCoordination/14(VINP_RrEDURealTMTq_Nm)
  DriverTqCoordination/3(VTQD_PreLoadHold_flg) -> VTQD_PreLoadHold_flg/1
  [VVMC_ADASActive_flg] -> PedalMapWhlTq/11(VVMC_ADASActive_flg)
  [VTQD_RDCActive_enum] -> Creep/18(VTQD_RDCActive_enum)
  VINP_ACCVehHoldReq_flg/1 -> [VINP_ACCVehHoldReq_flg]
  VVMC_APSReq_enum/1 -> [VVMC_APSReq_enum]
  [VVMC_APSReq_enum] -> Creep/19(VVMC_APSReq_enum)
  [VVMC_APSActive_flg] -> DriverTqCoordination/15(VVMC_APSActive_flg)
  [VVMC_ADASActive_flg] -> DriverTqCoordination/16(VVMC_ADASActive_flg)
  [VINP_ACCVehHoldReq_flg] -> DriverTqCoordination/17(VINP_ACCVehHoldReq_flg)
  [VINP_RrEDURealTMTq_Nm] -> Creep/21(VINP_RrEDURealTMTq_Nm)
  [VINP_FrEDURealTMTq_Nm] -> Creep/20(" VINP_FrEDURealTMTq_Nm")
  Creep/5(VTQD_CreepProtTqEn_flg) -> [VTQD_CreepProtTqEn_flg]
  [VTQD_CreepProtTqEn_flg] -> DriverTqCoordination/18(VTQD_CreepProtTqEn_flg)
  [VVMC_ActMaxSlideRate_pct] -> PedalMapWhlTq/12(VVMC_ActMaxSlideRate_pct)
  VVMC_LongAcc_Gps/1 -> [VVMC_LongAcc_Gps]
  VVMC_EstSlope_Deg/1 -> [VVMC_EstSlope_Deg]
  [VVMC_LongAcc_Gps] -> PedalMapWhlTq/14(VVMC_LongAcc_Gps)
  [VVMC_EstSlope_Deg] -> PedalMapWhlTq/13(VVMC_EstSlope_Deg)
  PedalMapWhlTq/3(VTQD_RegenTqLimitEn_flg) -> VTQD_RegenTqLimitEn_flg/1
  DriverTqCoordination/4(VTQD_PreLoadPreEn_flg) -> [VTQD_PreLoadPreEn_flg], VTQD_PreLoadPreEn_flg/1
  [VTQD_PreLoadPreEn_flg] -> Creep/22(VTQD_PreLoadPreEn_flg)
  [VVMC_EstSlope_Deg] -> Creep/23(VVMC_EstSlope_Deg)
  [VPMM_PwrSta_enum] -> Creep/24(VPMM_PwrSta_enum)
  [VTQD_TqTargetShaftSpd_rpm] -> DriverTqCoordination/19(VTQD_TqTargetShaftSpd_rpm)
  [VTQD_SysMode_enum] -> PedalMapWhlTq/15(VTQD_SysMode_enum)
  [VPMM_PwrSta_enum] -> PedalMapWhlTq/16(VPMM_PwrSta_enum)
  [VINP_SWCResUpSta_flg] -> PedalMapWhlTq/17(VINP_SWCResUpSta_flg)
  [task_time_s] -> PedalMapWhlTq/18(task_time_s)
  [VINP_VehSpeed_kph] -> PedalMapWhlTq/19(VINP_VehSpeed_kph)
  [VTQD_CreepPrLoadEnable_flg] -> PedalMapWhlTq/20(VTQD_CreepPrLoadEnable_flg)
  [VINP_BrkPedalPos_pct] -> PedalMapWhlTq/21(VINP_BrkPedalPos_pct)
  [VTQR_NoABSREDUWhlTqReq_Nm] -> PedalMapWhlTq/22(VTQR_NoABSREDUWhlTqReq_Nm)
  [VTQR_NoABSFEDUWhlTqReq_Nm] -> PedalMapWhlTq/23(VTQR_NoABSFEDUWhlTqReq_Nm)
  [VINP_FrPTCSActive_flg] -> PedalMapWhlTq/24(VINP_FrPTCSActive_flg)
  [VINP_RrPTCSActive_flg] -> PedalMapWhlTq/25(VINP_RrPTCSActive_flg)
  [VINP_ADASACCSta_enum] -> PedalMapWhlTq/26(VINP_ADASACCSta_enum)
  [VTQD_LowIdleAccPedal_flg] -> PedalMapWhlTq/27(VTQD_LowIdleAccPedal_flg)
  [VTQD_BrkSwSta_flg] -> PedalMapWhlTq/28(VTQD_BrkSwSta_flg)
  [VTQD_TqTargetShaftSpd_rpm] -> Creep/25(VTQD_TqTargetShaftSpd_rpm)
  [VTQD_APSReqTimer_s] -> Creep/26(VTQD_APSReqTimer_s)
  [VINP_EPBSta_enum] -> Creep/27(VINP_EPBSta_enum)
  Creep/6(VTQD_VehActSpd_kph) -> [VTQD_VehActSpd_kph], VTQD_VehActSpd_kph/1
  VINP_EPBSta_enum/1 -> [VINP_EPBSta_enum]
  VINP_RrPTCSActive_flg/1 -> [VINP_RrPTCSActive_flg]
  VTQD_SysMode_enum/1 -> [VTQD_SysMode_enum]
  VINP_BrkPedalPos_pct/1 -> [VINP_BrkPedalPos_pct]
  VINP_FrPTCSActive_flg/1 -> [VINP_FrPTCSActive_flg]
  VTQD_APSReqTimer_s/1 -> [VTQD_APSReqTimer_s]
  VTQR_NoABSFEDUWhlTqReq_Nm/1 -> [VTQR_NoABSFEDUWhlTqReq_Nm]
  VINP_ADASACCSta_enum/1 -> [VINP_ADASACCSta_enum]
  VTQR_NoABSREDUWhlTqReq_Nm/1 -> [VTQR_NoABSREDUWhlTqReq_Nm]
  VINP_SWCResUpSta_flg/1 -> [VINP_SWCResUpSta_flg]
  VPMM_PwrSta_enum/1 -> [VPMM_PwrSta_enum]
  [VTQD_PedalMapWhlTq_Nm] -> BOS/4(VTQD_PedalMapWhlTq_Nm)
  [VTQD_VehActSpd_kph] -> BOS/3(VTQD_VehActSpd_kph)
  Creep/7(VTQD_CreepBaseTqD_Nm) -> [VTQD_CreepBaseTqD_Nm], VTQD_CreepBaseTqD_Nm/1
  Creep/8(VTQD_CreepBaseTqR_Nm) -> [VTQD_CreepBaseTqR_Nm]
  [VTQD_BOSTq_Nm] -> DriverTqCoordination/5(VTQD_BOSTq_Nm)
  [VTQD_CreepBaseTqR_Nm] -> BOS/5(VTQD_CreepBaseTqR_Nm)
  [VTQD_CreepBaseTqD_Nm] -> BOS/6(VTQD_CreepBaseTqD_Nm)
  [VTQD_GearActualPosn_enum] -> BOS/7(VTQD_GearActualPosn_enum)
  VTQD_OPDHoldEnRel_flg/1 -> [VTQD_OPDHoldEnRel_flg]
  [VTQD_OPDHoldEnRel_flg] -> Creep/28(VTQD_OPDHoldEnRel_flg)
  [VVMC_APSActive_flg] -> BOS/8(VVMC_APSActive_flg)
  [VTQD_VehActSpd_kph] -> DriverTqCoordination/20(VTQD_VehActSpd_kph)
  [VTQD_ActAPSPosn_pct] -> Creep/29(VTQD_ActAPSPosn_pct)
  [VTQD_APSReqTimer_s] -> DriverTqCoordination/21(VTQD_APSReqTimer_s)
  [VTQD_CreepEnable_flg] -> DriverTqCoordination/22(VTQD_CreepEnable_flg)
  [VTQD_OPDHoldEnRel_flg] -> PedalMapWhlTq/29(VTQD_OPDHoldEnRel_flg)
  [VINP_SASAngle_Deg] -> PedalMapWhlTq/30(VINP_SASAngle_Deg)
  [VINP_YawRate_degps] -> PedalMapWhlTq/31(VINP_YawRate_degps)
  [VVMC_ActStESCYaw_degps] -> PedalMapWhlTq/32(VVMC_ActStESCYaw_degps)
  VINP_SASAngle_Deg/1 -> [VINP_SASAngle_Deg]
  VINP_YawRate_degps/1 -> [VINP_YawRate_degps]
  VVMC_ActStESCYaw_degps/1 -> [VVMC_ActStESCYaw_degps]
  VVMC_CAASActive_flg/1 -> [VVMC_CAASActive_flg]
  [VVMC_CAASActive_flg] -> Creep/30(VVMC_CAASActive_flg)
  [VVMC_LongAcc_Gps] -> DriverTqCoordination/6(VVMC_LongAcc_Gps)
  [VTQD_APSReqTimer_s] -> PedalMapWhlTq/33(VTQD_APSReqTimer_s)
  [VTQD_LowIdleAccPedal_flg] -> BOS/9(VTQD_LowIdleAccPedal_flg)
  [VTQD_OPDHoldActRelTq_Nm] -> PedalMapWhlTq/35(VTQD_OPDHoldActRelTq_Nm)
  [VTQD_VehActSpd_kph] -> PedalMapWhlTq/36(VTQD_VehActSpd_kph)
  Creep/9(VTQD_HighBPSPosn_flg) -> [VTQD_HighBPSPosn_flg]
  [VTQD_HighBPSPosn_flg] -> BOS/10(VTQD_HighBPSPosn_flg)
  [VTQD_BrkSwSta_flg] -> BOS/11(VTQD_BrkSwSta_flg)
  VTQD_OPDHoldActRelTq_Nm/1 -> [VTQD_OPDHoldActRelTq_Nm]
  [VINP_IVISnowModeCmd_flg] -> PedalMapWhlTq/37(VINP_IVISnowModeCmd_flg)
  VINP_IVISnowModeCmd_flg/1 -> [VINP_IVISnowModeCmd_flg]
  VVMC_LastADASWhlTqReq_Nm/1 -> [VVMC_LastADASWhlTqReq_Nm]  "VVMC_LastADASWhlTqReq_Nm"
  [VVMC_LastADASWhlTqReq_Nm] -> PedalMapWhlTq/34(VVMC_LastADASWhlTqReq_Nm)
  [VTQD_IVIRockModeEn_flg] -> PedalMapWhlTq/38(VTQD_IVIRockModeEn_flg)
  VTQD_IVIRockModeEn_flg/1 -> [VTQD_IVIRockModeEn_flg]
  PedalMapWhlTq/4(VTQD_PedAccTqEn_flg) -> VTQD_PedAccTqEn_flg/1, [VTQD_PedAccTqEn_flg]
  [VTQD_CreepEnable_flg] -> PedalMapWhlTq/39(VTQD_CreepEnable_flg)
  [VTQD_PedAccTqEn_flg] -> Creep/31(VTQD_PedAccTqEn_flg)
  [VTQR_RShaftSpdTqLimLow_flg] -> DriverTqCoordination/23(VTQR_RShaftSpdTqLimLow_flg)
  [VTQR_RTimerTqLimLow_flg] -> DriverTqCoordination/24(VTQR_RTimerTqLimLow_flg)
  [VTQR_FTimerTqLimLow_flg] -> DriverTqCoordination/26(VTQR_FTimerTqLimLow_flg)
  [VTQR_FShaftSpdTqLimLow_flg] -> DriverTqCoordination/25(VTQR_FShaftSpdTqLimLow_flg)
  [VTQD_ActAPSPosn_pct] -> DriverTqCoordination/27(VTQD_ActAPSPosn_pct)
  [VTQD_IVIRockModeEn_flg] -> DriverTqCoordination/28(VTQD_IVIRockModeEn_flg)
  [VINP_LFRawWhlSpeed_kph] -> DriverTqCoordination/29(VINP_LFRawWhlSpeed_kph)
  [VINP_LRRawWhlSpeed_kph] -> DriverTqCoordination/30(VINP_LRRawWhlSpeed_kph)
  [VINP_RFRawWhlSpeed_kph] -> DriverTqCoordination/31(VINP_RFRawWhlSpeed_kph)
  [VINP_RRRawWhlSpeed_kph] -> DriverTqCoordination/32(VINP_RRRawWhlSpeed_kph)
  [VTQD_FrShaftSpd_rpm] -> DriverTqCoordination/33(VTQD_FrShaftSpd_rpm)
  [VTQD_RrShaftSpd_rpm] -> DriverTqCoordination/34(VTQD_RrShaftSpd_rpm)
  VTQD_FrShaftSpd_rpm/1 -> [VTQD_FrShaftSpd_rpm]
  VINP_LRRawWhlSpeed_kph/1 -> [VINP_LRRawWhlSpeed_kph]
  VINP_RFRawWhlSpeed_kph/1 -> [VINP_RFRawWhlSpeed_kph]
  VINP_LFRawWhlSpeed_kph/1 -> [VINP_LFRawWhlSpeed_kph]
  VTQD_RrShaftSpd_rpm/1 -> [VTQD_RrShaftSpd_rpm]
  VTQR_RTimerTqLimLow_flg/1 -> [VTQR_RTimerTqLimLow_flg]
  VTQR_FShaftSpdTqLimLow_flg/1 -> [VTQR_FShaftSpdTqLimLow_flg]
  VINP_RRRawWhlSpeed_kph/1 -> [VINP_RRRawWhlSpeed_kph]
  VTQR_FTimerTqLimLow_flg/1 -> [VTQR_FTimerTqLimLow_flg]
  VTQR_RShaftSpdTqLimLow_flg/1 -> [VTQR_RShaftSpdTqLimLow_flg]
  DriverTqCoordination/5(VTQD_EscapModeTqLim_flg) -> VTQD_EscapModeTqLim_flg/1
  VINP_SWC2RCustomizeSta_flg/1 -> [VINP_SWC2RCustomizeSta_flg]
  [VINP_SWC2RCustomizeSta_flg] -> PedalMapWhlTq/40(VINP_SWC2RCustomizeSta_flg)
  Creep/10(VTQD_CreepTCSActive_flg) -> VTQD_CreepTCSActive_flg/1
  [VINP_RrPTCSActive_flg] -> Creep/33(VINP_RrPTCSActive_flg)
  [VINP_FrPTCSActive_flg] -> Creep/32(VINP_FrPTCSActive_flg)
  [VTQD_BrkSwSta_flg] -> Creep/34(VTQD_BrkSwSta_flg)
  VTQD_ActWhlSkipSta_enum/1 -> [VTQD_ActWhlSkipSta_enum]
  [VTQD_ActWhlSkipSta_enum] -> Creep/35(VTQD_ActWhlSkipSta_enum)
  VDDM_EPB1Err_flg/1 -> [VDDM_EPB1Err_flg]
  VDDM_ESC1Err_flg/1 -> [VDDM_ESC1Err_flg]
  VDDM_EPBSigErrCFS_flg/1 -> [VDDM_EPBSigErrCFS_flg]
  VDDM_ESC5Err_flg/1 -> [VDDM_ESC5Err_flg]
  [VDDM_EPB1Err_flg] -> Creep/36(VDDM_EPB1Err_flg)
  [VDDM_ESC1Err_flg] -> Creep/37(VDDM_ESC1Err_flg)
  [VDDM_ESC5Err_flg] -> Creep/38(VDDM_ESC5Err_flg)
  [VDDM_EPBSigErrCFS_flg] -> Creep/39(VDDM_EPBSigErrCFS_flg)
  VINP_ADASAEBSta_enum/1 -> [VINP_ADASAEBSta_enum]
  [VINP_ADASAEBSta_enum] -> DriverTqCoordination/35(VINP_ADASAEBSta_enum)
  [VTQD_ActWhlSkipSta_enum] -> DriverTqCoordination/36(VTQD_ActWhlSkipSta_enum)
  DriverTqCoordination/6(VTQD_FrPreloadTq_Nm) -> VTQD_FrPreloadTq_Nm/1
  DriverTqCoordination/7(VTQD_RrPreloadTq_Nm) -> VTQD_RrPreloadTq_Nm/1
  VDDM_MCUR1Err_flg/1 -> [VDDM_MCUR1Err_flg]
  VDDM_MCUF1Err_flg/1 -> [VDDM_MCUF1Err_flg]
  VDDM_VehMalfunLevel_enum/1 -> [VDDM_VehMalfunLevel_enum]
  [VDDM_VehMalfunLevel_enum] -> Creep/40(VDDM_VehMalfunLevel_enum)
  [VTQD_LimpHomeAct_flg] -> Creep/41(VTQD_LimpHomeAct_flg)
  [VDDM_MCUF1Err_flg] -> Creep/42(VDDM_MCUF1Err_flg)
  [VDDM_MCUR1Err_flg] -> Creep/43(VDDM_MCUR1Err_flg)
  [VDDM_VehMalfunLevel_enum] -> PedalMapWhlTq/41(VDDM_VehMalfunLevel_enum)
  [VTQD_LimpHomeAct_flg] -> BOS/12(VTQD_LimpHomeAct_flg)
  [VDDM_VehMalfunLevel_enum] -> DriverTqCoordination/37(VDDM_VehMalfunLevel_enum)
  PedalMapWhlTq/5(VTQD_SlideRegenLimTq_Nm) -> VTQD_SlideRegenLimTq_Nm/1
  [VDDM_VCURAPSErrLv2_flg] -> Creep/44(VDDM_VCURAPSErrLv2_flg)
  VDDM_VCURAPSErrLv2_flg/1 -> [VDDM_VCURAPSErrLv2_flg]

== system tqd/TQD/TorqueDemand/TorqueModule/ExtTqFuncHandShaking ==
  VPMM_PwrSta_enum : Inport
  VTQD_MCUReady4Ext_flg : Inport  Port=2
  VINP_HVBattErr_flg : Inport  Port=3
  VINP_DCDCFaultSta_enum : Inport  Port=4
  VINP_EPBErrSta_enum : Inport  Port=5
  VINP_DrDoorSW_flg : Inport  Port=6
  VINP_PsDoorSW_flg : Inport  Port=7
  VINP_RRDoorSW_flg : Inport  Port=8
  VINP_RLDoorSW_flg : Inport  Port=9
  VINP_HoodSW_flg : Inport  Port=10
  VINP_TailgateSW_flg : Inport  Port=11
  VDDM_Shifter1Err_flg : Inport  Port=12
  VDDM_ShifterSigErrCFS_flg : Inport  Port=13
  VTQD_LimpHomeAct_flg : Inport  Port=14
  VDDM_EPBSigErrCFS_flg : Inport  Port=15
  VDDM_4D2CErr_flg : Inport  Port=16
  VDDM_EPB1Err_flg : Inport  Port=17
  VVMC_APSActive_flg : Inport  Port=18
  Constant1 : Constant  Value=KTQD_ExtTqAllow_flg_ovrdflg
  Constant10 : Constant  Value=TRUE
  Constant11 : Constant  Value=FALSE
  Constant12 : Constant  Value=ENUM_EPBERROR_NORMAL
  Constant13 : Constant  Value=KTQD_ExtDoorAllow_flg_ovrdflg
  Constant14 : Constant  Value=KTQD_ExtDoorAllow_flg_ovrdval
  Constant15 : Constant  Value=ENUM_POWERSTA_READY
  Constant16 : Constant  Value=ENUM_POWERSTA_ON
  Constant17 : Constant  Value=ENUM_POWERSTA_READY
  Constant18 : Constant  Value=ENUM_POWERSTA_ON
  Constant19 : Constant  Value=KTQD_PassAPSActive_flg_ovrdflg
  Constant2 : Constant  Commented=on  Value=ENUM_DCDCFAULTSTA_WORKING
  Constant20 : Constant  Value=KTQD_PassAPSActive_flg_ovrdflg
  Constant21 : Constant  Value=KTQD_PassAPSActive_flg_ovrdval
  Constant22 : Constant  Value=KTQD_PassAPSActive_flg_ovrdval
  Constant3 : Constant  Value=KTQD_ExtTqAllow_flg_ovrdval
  Constant4 : Constant  Commented=on  Value=ENUM_DCDCFAULTSTA_WORKING
  Constant5 : Constant  Commented=on  Value=ENUM_EPBERROR_NORMAL
  Constant6 : Constant  Value=KTQD_ExtShftAllow_flg_ovrdflg
  Constant7 : Constant  Value=KTQD_ExtShftAllow_flg_ovrdval
  Constant8 : Constant  Value=TRUE
  Constant9 : Constant  Value=FALSE
  Equal1 : RelationalOperator  Commented=on  Operator===  OutDataTypeStr=boolean  RndMeth=Simplest
  Equal2 : RelationalOperator  Commented=on  Operator===  OutDataTypeStr=boolean  RndMeth=Simplest
  Equal3 : RelationalOperator  Commented=on  Operator===  OutDataTypeStr=boolean  RndMeth=Simplest
  Equal{4..8} (5 alike) : RelationalOperator  Operator===  OutDataTypeStr=boolean  RndMeth=Simplest
  From1 : From  Commented=on  GotoTag=VTQD_MCUReady4Ext_flg
  From2 : From  Commented=on  GotoTag=VINP_HVBattErr_flg
  From3 : From  Commented=on  GotoTag=VINP_DCDCFaultSta_enum
  From4 : From  Commented=on  GotoTag=VTQD_MCUReady4Ext_flg
  From5 : From  Commented=on  GotoTag=VINP_HVBattErr_flg
  From6 : From  Commented=on  GotoTag=VINP_DCDCFaultSta_enum
  From8 : From  Commented=on  GotoTag=VINP_EPBErrSta_enum
  LiuzgSwitch{1..7} (7 alike) : Switch  Criteria=u2 ~= 0
      settings: AttributesFormatString=<%<Criteria>>
  Logical Operator : Logic  Commented=on  Operator=NOT  AllPortsSameDT=off  OutDataTypeStr=boolean
  Logical Operator1 : Logic  Commented=on  Operator=NOT  AllPortsSameDT=off  OutDataTypeStr=boolean
  Logical Operator{4..7,9..10} (6 alike) : Logic  Operator=NOT  AllPortsSameDT=off  OutDataTypeStr=boolean
  Logical Operator11 : Logic  AllPortsSameDT=off  OutDataTypeStr=boolean
  Logical Operator12 : Logic  AllPortsSameDT=off  OutDataTypeStr=boolean
  Logical Operator2 : Logic  Operator=OR  AllPortsSameDT=off  OutDataTypeStr=boolean
  Logical Operator3 : Logic  Operator=OR  AllPortsSameDT=off  OutDataTypeStr=boolean
  Logical Operator8 : Logic  Inputs=3  AllPortsSameDT=off  OutDataTypeStr=boolean
  NOT{,1..6} (7 alike) : Logic  Operator=NOT  AllPortsSameDT=off  OutDataTypeStr=boolean
  OR : Logic  AllPortsSameDT=off  OutDataTypeStr=boolean
  OR1 : Logic  Inputs=5  AllPortsSameDT=off  OutDataTypeStr=boolean
  OR2 : Logic  Inputs=7  AllPortsSameDT=off  OutDataTypeStr=boolean
  Terminator : Terminator
  Terminator1 : Terminator
  Terminator2 : Terminator
  VTQD_ExternalTqAllow_flg : Outport
  VTQD_ExtShftAllow_flg : Outport  Port=2
  VTQD_ExtDoorAllow_flg : Outport  Port=3
  wires:
  VTQD_MCUReady4Ext_flg/1 -> [VTQD_MCUReady4Ext_flg]
  Constant2/1 -> Equal2/2
  From3/1 -> Equal2/1
  From2/1 -> Logical Operator/1
  VINP_HVBattErr_flg/1 -> [VINP_HVBattErr_flg]
  VINP_DCDCFaultSta_enum/1 -> [VINP_DCDCFaultSta_enum]
  VPMM_PwrSta_enum/1 -> [VPMM_PwrSta_enum]
  LiuzgSwitch1/1 -> VTQD_ExternalTqAllow_flg/1  "VTQD_ExternalTqAllow_flg"
  Constant1/1 -> LiuzgSwitch1/2
  Constant3/1 -> LiuzgSwitch1/1
  VINP_EPBErrSta_enum/1 -> [VINP_EPBErrSta_enum]
  Constant5/1 -> Equal3/2
  LiuzgSwitch2/1 -> VTQD_ExtShftAllow_flg/1  "VTQD_ExtShftAllow_flg"
  Constant4/1 -> Equal1/2
  From5/1 -> Logical Operator1/1
  From8/1 -> Equal3/1
  From6/1 -> Equal1/1
  Constant6/1 -> LiuzgSwitch2/2
  Constant7/1 -> LiuzgSwitch2/1
  Constant8/1 -> LiuzgSwitch3/1
  Constant9/1 -> LiuzgSwitch3/3
  Constant11/1 -> LiuzgSwitch4/3
  Constant10/1 -> LiuzgSwitch4/1
  OR/1 -> LiuzgSwitch4/2
  LiuzgSwitch5/1 -> VTQD_ExtDoorAllow_flg/1  "VTQD_ExtDoorAllow_flg"
  Constant14/1 -> LiuzgSwitch5/1
  Constant13/1 -> LiuzgSwitch5/2
  NOT5/1 -> OR2/6
  NOT4/1 -> OR2/5
  OR2/1 -> LiuzgSwitch5/3
  NOT2/1 -> OR2/3
  NOT/1 -> OR2/1
  NOT1/1 -> OR2/2
  NOT3/1 -> OR2/4
  [VINP_DrDoorSW_flg] -> NOT/1
  VINP_TailgateSW_flg/1 -> [VINP_TailgateSW_flg]
  VINP_RRDoorSW_flg/1 -> [VINP_RRDoorSW_flg]
  VINP_RLDoorSW_flg/1 -> [VINP_RLDoorSW_flg]
  VINP_HoodSW_flg/1 -> [VINP_HoodSW_flg]
  VINP_DrDoorSW_flg/1 -> [VINP_DrDoorSW_flg]
  VINP_PsDoorSW_flg/1 -> [VINP_PsDoorSW_flg]
  [VINP_PsDoorSW_flg] -> NOT1/1
  [VINP_RRDoorSW_flg] -> NOT2/1
  [VINP_RLDoorSW_flg] -> NOT3/1
  [VINP_HoodSW_flg] -> NOT4/1
  [VINP_TailgateSW_flg] -> NOT5/1
  Equal8/1 -> Logical Operator3/2
  Equal7/1 -> Logical Operator3/1
  [VPMM_PwrSta_enum] -> Equal8/1
  Constant17/1 -> Equal7/2
  [VPMM_PwrSta_enum] -> Equal7/1
  Logical Operator3/1 -> OR/1
  Constant18/1 -> Equal8/2
  VDDM_Shifter1Err_flg/1 -> [VDDM_Shifter1Err_flg]
  VDDM_ShifterSigErrCFS_flg/1 -> [VDDM_ShifterSigErrCFS_flg]
  VDDM_EPB1Err_flg/1 -> [VDDM_EPB1Err_flg]
  VTQD_LimpHomeAct_flg/1 -> [VTQD_LimpHomeAct_flg]
  VDDM_4D2CErr_flg/1 -> [VDDM_4D2CErr_flg]
  VDDM_EPBSigErrCFS_flg/1 -> [VDDM_EPBSigErrCFS_flg]
  [VINP_HVBattErr_flg] -> Terminator1/1
  [VINP_DCDCFaultSta_enum] -> Terminator2/1
  [VTQD_MCUReady4Ext_flg] -> Terminator/1
  [VTQD_LimpHomeAct_flg] -> Logical Operator6/1
  Logical Operator6/1 -> OR/2
  Logical Operator10/1 -> Logical Operator8/2
  [VPMM_PwrSta_enum] -> Equal6/1
  [VDDM_EPBSigErrCFS_flg] -> Logical Operator9/1
  [VINP_EPBErrSta_enum] -> Equal4/1
  Logical Operator2/1 -> OR1/1
  Equal6/1 -> Logical Operator2/2
  Equal4/1 -> Logical Operator8/3
  Constant16/1 -> Equal6/2
  [VDDM_Shifter1Err_flg] -> Logical Operator4/1
  Constant12/1 -> Equal4/2
  Logical Operator5/1 -> OR1/5
  Constant15/1 -> Equal5/2
  Logical Operator4/1 -> OR1/4
  Logical Operator9/1 -> Logical Operator8/1
  [VPMM_PwrSta_enum] -> Equal5/1
  [VTQD_LimpHomeAct_flg] -> Logical Operator7/1
  [VDDM_EPB1Err_flg] -> Logical Operator10/1
  Equal5/1 -> Logical Operator2/1
  Logical Operator8/1 -> OR1/2
  Logical Operator7/1 -> OR1/3
  [VDDM_ShifterSigErrCFS_flg] -> Logical Operator5/1
  OR1/1 -> LiuzgSwitch3/2
  [VDDM_4D2CErr_flg] -> NOT6/1
  NOT6/1 -> OR2/7
  Constant19/1 -> Logical Operator11/2
  Constant21/1 -> LiuzgSwitch6/1
  Logical Operator11/1 -> LiuzgSwitch6/2
  [VVMC_APSActive_flg] -> Logical Operator11/1
  LiuzgSwitch4/1 -> LiuzgSwitch6/3
  LiuzgSwitch6/1 -> LiuzgSwitch1/3
  [VVMC_APSActive_flg] -> Logical Operator12/1
  Constant20/1 -> Logical Operator12/2
  Constant22/1 -> LiuzgSwitch7/1
  Logical Operator12/1 -> LiuzgSwitch7/2
  LiuzgSwitch3/1 -> LiuzgSwitch7/3
  LiuzgSwitch7/1 -> LiuzgSwitch2/3
  VVMC_APSActive_flg/1 -> [VVMC_APSActive_flg]
